simulink model "train_detection"  (R2024b)
settings: Solver=FixedStepAuto  StartTime=0.0  StopTime=simDuration  FixedStep=0.01  RelTol=1e-3
InitFcn:
  | breakp=[-1, -0.9, -0.8, -0.6, -0.4, -0.2, -0.1, 0, 0.1, 0.2, 0.4, 0.6, 0.8, 1];
  | 
  | splinenew =[-1, -0.92, -0.8, -0.50, -0.28, -0.12, -0.05, 0, 0.005, 0.01, 0.02, 0.025,0.03,0.035];
undefined symbols (not defined in the file or in its folder): Discrete, K, qbreak, Time
libraries: simulink x25, ctrlSharedLib x4, dspfdesign x2
(part 2 of 2)

== system train_detection/RIGHT_LEG/Pos and Vel normalized/Subsystem ==
  Angle : Inport
  Trigger : TriggerPort  VariantControl=Variant  PortDimensions=1
  Angle_min : Outport
  wires:
  Angle/1 -> Angle_min/1

== system train_detection/RIGHT_LEG/Pos and Vel normalized/Subsystem1 ==
  Velocity : Inport
  Trigger : TriggerPort  VariantControl=Variant  PortDimensions=1
  Vel_max : Outport
  wires:
  Velocity/1 -> Vel_max/1

== system train_detection/RIGHT_LEG/Pos and Vel normalized/Subsystem2 ==
  angle : Inport
  Trigger : TriggerPort  VariantControl=Variant  PortDimensions=1
  Angle_max : Outport
  wires:
  angle/1 -> Angle_max/1

== system train_detection/RIGHT_LEG/Pos and Vel normalized/Subsystem3 ==
  Velocity : Inport
  Trigger : TriggerPort  VariantControl=Variant  PortDimensions=1
  Vel_min : Outport
  wires:
  Velocity/1 -> Vel_min/1

== system train_detection/RIGHT_LEG/Pos and Vel normalized/Subsystem4 ==
  Clock : Inport
  angle : Inport  Port=2
  Trigger : TriggerPort  VariantControl=Variant  PortDimensions=1
  If : If  ShowElse=off
  If Action Subsystem : Subsystem  TreatAsAtomicUnit=on
  Angle_max : Outport
  wires:
  If/1 -> If Action Subsystem/Action
  angle/1 -> If Action Subsystem/2(angle), If/1
  If Action Subsystem/1(Angle_max) -> Angle_max/1  "angle_max"
  Clock/1 -> If Action Subsystem/1(Clock)  "clock"

== system train_detection/RIGHT_LEG/Pos and Vel normalized/Subsystem5 ==
  Angle : Inport
  Clock : Inport  Port=2
  Trigger : TriggerPort  VariantControl=Variant  PortDimensions=1
  If : If  IfExpression=u1 < 0  ShowElse=off
  If Action Subsystem : Subsystem  TreatAsAtomicUnit=on
  Angle_min : Outport
  wires:
  If/1 -> If Action Subsystem/Action
  Angle/1 -> If Action Subsystem/1(Angle), If/1
  If Action Subsystem/1(Angle_min) -> Angle_min/1  "angle_min"
  Clock/1 -> If Action Subsystem/2(Clock)  "clock"

== system train_detection/RIGHT_LEG/Pos and Vel normalized/Subsystem6 ==
  Velocity : Inport
  Clock : Inport  Port=2
  Trigger : TriggerPort  VariantControl=Variant  PortDimensions=1
  If : If  IfExpression=u1 < 0  ShowElse=off
  If Action Subsystem : Subsystem  TreatAsAtomicUnit=on
  Vel_min : Outport
  wires:
  If Action Subsystem/1(Vel_min) -> Vel_min/1  "vel_min"
  If/1 -> If Action Subsystem/Action
  Velocity/1 -> If Action Subsystem/1(Velocity), If/1
  Clock/1 -> If Action Subsystem/2(Clock)  "clock"

== system train_detection/RIGHT_LEG/Pos and Vel normalized/Subsystem7 ==
  Velocity : Inport
  Clock : Inport  Port=2
  Trigger : TriggerPort  VariantControl=Variant  PortDimensions=1
  If : If  ShowElse=off
  If Action Subsystem : Subsystem  TreatAsAtomicUnit=on
  Vel_max : Outport
  wires:
  If/1 -> If Action Subsystem/Action
  Velocity/1 -> If Action Subsystem/1(Velocity), If/1
  Clock/1 -> If Action Subsystem/2(Clock)  "clock"
  If Action Subsystem/1(Vel_max) -> Vel_max/1  "vel_max"

== system train_detection/RIGHT_LEG/Pos normalized/Subsystem ==
  Angle : Inport
  Clock : Inport  Port=2
  Trigger : TriggerPort  VariantControl=Variant  PortDimensions=1
  If : If  IfExpression=u1 < 0  ShowElse=off
  If Action Subsystem : Subsystem  TreatAsAtomicUnit=on
  Angle_min : Outport
  wires:
  If Action Subsystem/1(Angle_min) -> Angle_min/1  "angle_min"
  Clock/1 -> If Action Subsystem/2(Clock)  "clock"
  If/1 -> If Action Subsystem/Action
  Angle/1 -> If Action Subsystem/1(Angle), If/1

== system train_detection/RIGHT_LEG/Pos normalized/Subsystem2 ==
  Clock : Inport
  angle : Inport  Port=2
  Trigger : TriggerPort  VariantControl=Variant  PortDimensions=1
  If : If  ShowElse=off
  If Action Subsystem : Subsystem  TreatAsAtomicUnit=on
  Angle_out : Outport
  wires:
  If Action Subsystem/1(Angle_out) -> Angle_out/1  "angle_out"
  angle/1 -> If Action Subsystem/2(angle), If/1
  If/1 -> If Action Subsystem/Action
  Clock/1 -> If Action Subsystem/1(Clock)  "clock"

== system train_detection/RIGHT_LEG/Vel normalized/Subsystem1 ==
  Velocity : Inport
  Clock : Inport  Port=2
  Trigger : TriggerPort  VariantControl=Variant  PortDimensions=1
  If : If  ShowElse=off
  If Action Subsystem : Subsystem  TreatAsAtomicUnit=on
  Vel_max : Outport
  wires:
  If Action Subsystem/1(Vel_max) -> Vel_max/1  "vel_max"
  Velocity/1 -> If/1, If Action Subsystem/1(Velocity)
  If/1 -> If Action Subsystem/Action
  Clock/1 -> If Action Subsystem/2(Clock)  "clock"

== system train_detection/RIGHT_LEG/Vel normalized/Subsystem3 ==
  Velocity : Inport
  Clock : Inport  Port=2
  Trigger : TriggerPort  VariantControl=Variant  PortDimensions=1
  If : If  IfExpression=u1 < 0  ShowElse=off
  If Action Subsystem : Subsystem  TreatAsAtomicUnit=on
  Vel_min : Outport
  wires:
  If Action Subsystem/1(Vel_min) -> Vel_min/1  "vel_min"
  Clock/1 -> If Action Subsystem/2(Clock)  "clock"
  Velocity/1 -> If Action Subsystem/1(Velocity), If/1
  If/1 -> If Action Subsystem/Action

== system train_detection/RIGHT_LEG1/Pos and Vel normalized/Subsystem ==
  Angle : Inport
  Trigger : TriggerPort  VariantControl=Variant  PortDimensions=1
  Angle_min : Outport
  wires:
  Angle/1 -> Angle_min/1

== system train_detection/RIGHT_LEG1/Pos and Vel normalized/Subsystem1 ==
  Velocity : Inport
  Trigger : TriggerPort  VariantControl=Variant  PortDimensions=1
  Vel_max : Outport
  wires:
  Velocity/1 -> Vel_max/1

== system train_detection/RIGHT_LEG1/Pos and Vel normalized/Subsystem2 ==
  angle : Inport
  Trigger : TriggerPort  VariantControl=Variant  PortDimensions=1
  Angle_max : Outport
  wires:
  angle/1 -> Angle_max/1

== system train_detection/RIGHT_LEG1/Pos and Vel normalized/Subsystem3 ==
  Velocity : Inport
  Trigger : TriggerPort  VariantControl=Variant  PortDimensions=1
  Vel_min : Outport
  wires:
  Velocity/1 -> Vel_min/1

== system train_detection/RIGHT_LEG1/Pos and Vel normalized/Subsystem4 ==
  Clock : Inport
  angle : Inport  Port=2
  Trigger : TriggerPort  VariantControl=Variant  PortDimensions=1
  If : If  ShowElse=off
  If Action Subsystem : Subsystem  TreatAsAtomicUnit=on
  Angle_max : Outport
  wires:
  If/1 -> If Action Subsystem/Action
  angle/1 -> If Action Subsystem/2(angle), If/1
  If Action Subsystem/1(Angle_max) -> Angle_max/1  "angle_max"
  Clock/1 -> If Action Subsystem/1(Clock)  "clock"

== system train_detection/RIGHT_LEG1/Pos and Vel normalized/Subsystem5 ==
  Angle : Inport
  Clock : Inport  Port=2
  Trigger : TriggerPort  VariantControl=Variant  PortDimensions=1
  If : If  IfExpression=u1 < 0  ShowElse=off
  If Action Subsystem : Subsystem  TreatAsAtomicUnit=on
  Angle_min : Outport
  wires:
  If/1 -> If Action Subsystem/Action
  Angle/1 -> If Action Subsystem/1(Angle), If/1
  If Action Subsystem/1(Angle_min) -> Angle_min/1  "angle_min"
  Clock/1 -> If Action Subsystem/2(Clock)  "clock"

== system train_detection/RIGHT_LEG1/Pos and Vel normalized/Subsystem6 ==
  Velocity : Inport
  Clock : Inport  Port=2
  Trigger : TriggerPort  VariantControl=Variant  PortDimensions=1
  If : If  IfExpression=u1 < 0  ShowElse=off
  If Action Subsystem : Subsystem  TreatAsAtomicUnit=on
  Vel_min : Outport
  wires:
  If Action Subsystem/1(Vel_min) -> Vel_min/1  "vel_min"
  If/1 -> If Action Subsystem/Action
  Velocity/1 -> If Action Subsystem/1(Velocity), If/1
  Clock/1 -> If Action Subsystem/2(Clock)  "clock"

== system train_detection/RIGHT_LEG1/Pos and Vel normalized/Subsystem7 ==
  Velocity : Inport
  Clock : Inport  Port=2
  Trigger : TriggerPort  VariantControl=Variant  PortDimensions=1
  If : If  ShowElse=off
  If Action Subsystem : Subsystem  TreatAsAtomicUnit=on
  Vel_max : Outport
  wires:
  If/1 -> If Action Subsystem/Action
  Velocity/1 -> If Action Subsystem/1(Velocity), If/1
  Clock/1 -> If Action Subsystem/2(Clock)  "clock"
  If Action Subsystem/1(Vel_max) -> Vel_max/1  "vel_max"

== system train_detection/RIGHT_LEG1/Pos normalized/Subsystem ==
  Angle : Inport
  Clock : Inport  Port=2
  Trigger : TriggerPort  VariantControl=Variant  PortDimensions=1
  If : If  IfExpression=u1 < 0  ShowElse=off
  If Action Subsystem : Subsystem  TreatAsAtomicUnit=on
  Angle_min : Outport
  wires:
  If Action Subsystem/1(Angle_min) -> Angle_min/1  "angle_min"
  Clock/1 -> If Action Subsystem/2(Clock)  "clock"
  If/1 -> If Action Subsystem/Action
  Angle/1 -> If Action Subsystem/1(Angle), If/1

== system train_detection/RIGHT_LEG1/Pos normalized/Subsystem2 ==
  Clock : Inport
  angle : Inport  Port=2
  Trigger : TriggerPort  VariantControl=Variant  PortDimensions=1
  If : If  ShowElse=off
  If Action Subsystem : Subsystem  TreatAsAtomicUnit=on
  Angle_out : Outport
  wires:
  If Action Subsystem/1(Angle_out) -> Angle_out/1  "angle_out"
  angle/1 -> If Action Subsystem/2(angle), If/1
  If/1 -> If Action Subsystem/Action
  Clock/1 -> If Action Subsystem/1(Clock)  "clock"

== system train_detection/RIGHT_LEG1/Vel normalized/Subsystem1 ==
  Velocity : Inport
  Clock : Inport  Port=2
  Trigger : TriggerPort  VariantControl=Variant  PortDimensions=1
  If : If  ShowElse=off
  If Action Subsystem : Subsystem  TreatAsAtomicUnit=on
  Vel_max : Outport
  wires:
  If Action Subsystem/1(Vel_max) -> Vel_max/1  "vel_max"
  Velocity/1 -> If/1, If Action Subsystem/1(Velocity)
  If/1 -> If Action Subsystem/Action
  Clock/1 -> If Action Subsystem/2(Clock)  "clock"

== system train_detection/RIGHT_LEG1/Vel normalized/Subsystem3 ==
  Velocity : Inport
  Clock : Inport  Port=2
  Trigger : TriggerPort  VariantControl=Variant  PortDimensions=1
  If : If  IfExpression=u1 < 0  ShowElse=off
  If Action Subsystem : Subsystem  TreatAsAtomicUnit=on
  Vel_min : Outport
  wires:
  If Action Subsystem/1(Vel_min) -> Vel_min/1  "vel_min"
  Clock/1 -> If Action Subsystem/2(Clock)  "clock"
  Velocity/1 -> If Action Subsystem/1(Velocity), If/1
  If/1 -> If Action Subsystem/Action

== system train_detection/LEFT LEG/Pos and Vel normalized/Subsystem4/If Action Subsystem ==
  Clock : Inport
  angle : Inport  Port=2
  Action Port : ActionPort
  Compare To Constant1 : simulink/Logic and Bit Operations/Compare To Constant  relop=>=  const=0.3  OutDataTypeStr=boolean
  Enabled Subsystem : Subsystem  TreatAsAtomicUnit=on
  Memory : Memory  InheritSampleTime=on
  Subtract : Sum  Inputs=+-
  Zero-Order Hold : ZeroOrderHold  SampleTime=-1
  Angle_max : Outport
  wires:
  Subtract/1 -> Compare To Constant1/1  "diff"
  Compare To Constant1/1 -> Enabled Subsystem/Enable  "enable"
  Enabled Subsystem/1(angle_out) -> Angle_max/1  "angle_out"
  angle/1 -> Enabled Subsystem/1(angle_in)
  Clock/1 -> Zero-Order Hold/1  "clock"
  Zero-Order Hold/1 -> Subtract/1, Memory/1  "clock_ZOH"
  Memory/1 -> Subtract/2  "clock_memory"

== system train_detection/LEFT LEG/Pos and Vel normalized/Subsystem5/If Action Subsystem ==
  Angle : Inport
  Clock : Inport  Port=2
  Action Port : ActionPort
  Compare To Constant1 : simulink/Logic and Bit Operations/Compare To Constant  relop=>=  const=0.3  OutDataTypeStr=boolean
  Enabled Subsystem : Subsystem  TreatAsAtomicUnit=on
  Memory : Memory  InheritSampleTime=on
  Subtract : Sum  Inputs=+-
  Zero-Order Hold : ZeroOrderHold  SampleTime=-1
  Angle_min : Outport
  wires:
  Memory/1 -> Subtract/2  "clock_memory"
  Zero-Order Hold/1 -> Subtract/1, Memory/1  "clock_ZOH"
  Enabled Subsystem/1(angle_out) -> Angle_min/1  "angle_out"
  Compare To Constant1/1 -> Enabled Subsystem/Enable  "enable"
  Clock/1 -> Zero-Order Hold/1  "clock"
  Subtract/1 -> Compare To Constant1/1  "diff"
  Angle/1 -> Enabled Subsystem/1(angle_in)

== system train_detection/LEFT LEG/Pos and Vel normalized/Subsystem6/If Action Subsystem ==
  Velocity : Inport
  Clock : Inport  Port=2
  Action Port : ActionPort
  Compare To Constant1 : simulink/Logic and Bit Operations/Compare To Constant  relop=>=  const=0.3  OutDataTypeStr=boolean
  Enabled Subsystem : Subsystem  TreatAsAtomicUnit=on
  Memory : Memory  InheritSampleTime=on
  Subtract : Sum  Inputs=+-
  Zero-Order Hold : ZeroOrderHold  SampleTime=-1
  Vel_min : Outport
  wires:
  Enabled Subsystem/1(vel_out) -> Vel_min/1  "angle_out"
  Memory/1 -> Subtract/2  "clock_memory"
  Velocity/1 -> Enabled Subsystem/1(vel_in)
  Zero-Order Hold/1 -> Subtract/1, Memory/1  "clock_ZOH"
  Clock/1 -> Zero-Order Hold/1  "clock"
  Subtract/1 -> Compare To Constant1/1  "diff"
  Compare To Constant1/1 -> Enabled Subsystem/Enable  "enable"

== system train_detection/LEFT LEG/Pos and Vel normalized/Subsystem7/If Action Subsystem ==
  Velocity : Inport
  Clock : Inport  Port=2
  Action Port : ActionPort
  Compare To Constant1 : simulink/Logic and Bit Operations/Compare To Constant  relop=>=  const=0.3  OutDataTypeStr=boolean
  Enabled Subsystem : Subsystem  TreatAsAtomicUnit=on
  Memory : Memory  InheritSampleTime=on
  Subtract : Sum  Inputs=+-
  Zero-Order Hold : ZeroOrderHold  SampleTime=-1
  Vel_max : Outport
  wires:
  Memory/1 -> Subtract/2  "clock_memory"
  Compare To Constant1/1 -> Enabled Subsystem/Enable  "enable"
  Clock/1 -> Zero-Order Hold/1  "clock"
  Zero-Order Hold/1 -> Subtract/1, Memory/1  "clock_ZOH"
  Enabled Subsystem/1(vel_out) -> Vel_max/1  "angle_out"
  Subtract/1 -> Compare To Constant1/1  "diff"
  Velocity/1 -> Enabled Subsystem/1(vel_in)

== system train_detection/LEFT LEG1/Pos and Vel normalized/Subsystem4/If Action Subsystem ==
  Clock : Inport
  angle : Inport  Port=2
  Action Port : ActionPort
  Compare To Constant1 : simulink/Logic and Bit Operations/Compare To Constant  relop=>=  const=0.3  OutDataTypeStr=boolean
  Enabled Subsystem : Subsystem  TreatAsAtomicUnit=on
  Memory : Memory  InheritSampleTime=on
  Subtract : Sum  Inputs=+-
  Zero-Order Hold : ZeroOrderHold  SampleTime=-1
  Angle_max : Outport
  wires:
  Subtract/1 -> Compare To Constant1/1  "diff"
  Compare To Constant1/1 -> Enabled Subsystem/Enable  "enable"
  Enabled Subsystem/1(angle_out) -> Angle_max/1  "angle_out"
  angle/1 -> Enabled Subsystem/1(angle_in)
  Clock/1 -> Zero-Order Hold/1  "clock"
  Zero-Order Hold/1 -> Subtract/1, Memory/1  "clock_ZOH"
  Memory/1 -> Subtract/2  "clock_memory"

== system train_detection/LEFT LEG1/Pos and Vel normalized/Subsystem5/If Action Subsystem ==
  Angle : Inport
  Clock : Inport  Port=2
  Action Port : ActionPort
  Compare To Constant1 : simulink/Logic and Bit Operations/Compare To Constant  relop=>=  const=0.3  OutDataTypeStr=boolean
  Enabled Subsystem : Subsystem  TreatAsAtomicUnit=on
  Memory : Memory  InheritSampleTime=on
  Subtract : Sum  Inputs=+-
  Zero-Order Hold : ZeroOrderHold  SampleTime=-1
  Angle_min : Outport
  wires:
  Memory/1 -> Subtract/2  "clock_memory"
  Zero-Order Hold/1 -> Subtract/1, Memory/1  "clock_ZOH"
  Enabled Subsystem/1(angle_out) -> Angle_min/1  "angle_out"
  Compare To Constant1/1 -> Enabled Subsystem/Enable  "enable"
  Clock/1 -> Zero-Order Hold/1  "clock"
  Subtract/1 -> Compare To Constant1/1  "diff"
  Angle/1 -> Enabled Subsystem/1(angle_in)

== system train_detection/LEFT LEG1/Pos and Vel normalized/Subsystem6/If Action Subsystem ==
  Velocity : Inport
  Clock : Inport  Port=2
  Action Port : ActionPort
  Compare To Constant1 : simulink/Logic and Bit Operations/Compare To Constant  relop=>=  const=0.3  OutDataTypeStr=boolean
  Enabled Subsystem : Subsystem  TreatAsAtomicUnit=on
  Memory : Memory  InheritSampleTime=on
  Subtract : Sum  Inputs=+-
  Zero-Order Hold : ZeroOrderHold  SampleTime=-1
  Vel_min : Outport
  wires:
  Enabled Subsystem/1(vel_out) -> Vel_min/1  "angle_out"
  Memory/1 -> Subtract/2  "clock_memory"
  Velocity/1 -> Enabled Subsystem/1(vel_in)
  Zero-Order Hold/1 -> Subtract/1, Memory/1  "clock_ZOH"
  Clock/1 -> Zero-Order Hold/1  "clock"
  Subtract/1 -> Compare To Constant1/1  "diff"
  Compare To Constant1/1 -> Enabled Subsystem/Enable  "enable"

== system train_detection/LEFT LEG1/Pos and Vel normalized/Subsystem7/If Action Subsystem ==
  Velocity : Inport
  Clock : Inport  Port=2
  Action Port : ActionPort
  Compare To Constant1 : simulink/Logic and Bit Operations/Compare To Constant  relop=>=  const=0.3  OutDataTypeStr=boolean
  Enabled Subsystem : Subsystem  TreatAsAtomicUnit=on
  Memory : Memory  InheritSampleTime=on
  Subtract : Sum  Inputs=+-
  Zero-Order Hold : ZeroOrderHold  SampleTime=-1
  Vel_max : Outport
  wires:
  Memory/1 -> Subtract/2  "clock_memory"
  Compare To Constant1/1 -> Enabled Subsystem/Enable  "enable"
  Clock/1 -> Zero-Order Hold/1  "clock"
  Zero-Order Hold/1 -> Subtract/1, Memory/1  "clock_ZOH"
  Enabled Subsystem/1(vel_out) -> Vel_max/1  "angle_out"
  Subtract/1 -> Compare To Constant1/1  "diff"
  Velocity/1 -> Enabled Subsystem/1(vel_in)

== system train_detection/RIGHT_LEG/Pos and Vel normalized/Subsystem4/If Action Subsystem ==
  Clock : Inport
  angle : Inport  Port=2
  Action Port : ActionPort
  Compare To Constant1 : simulink/Logic and Bit Operations/Compare To Constant  relop=>=  const=0.3  OutDataTypeStr=boolean
  Enabled Subsystem : Subsystem  TreatAsAtomicUnit=on
  Memory : Memory  InheritSampleTime=on
  Subtract : Sum  Inputs=+-
  Zero-Order Hold : ZeroOrderHold  SampleTime=-1
  Angle_max : Outport
  wires:
  Subtract/1 -> Compare To Constant1/1  "diff"
  Compare To Constant1/1 -> Enabled Subsystem/Enable  "enable"
  Enabled Subsystem/1(angle_out) -> Angle_max/1  "angle_out"
  angle/1 -> Enabled Subsystem/1(angle_in)
  Clock/1 -> Zero-Order Hold/1  "clock"
  Zero-Order Hold/1 -> Subtract/1, Memory/1  "clock_ZOH"
  Memory/1 -> Subtract/2  "clock_memory"

== system train_detection/RIGHT_LEG/Pos and Vel normalized/Subsystem5/If Action Subsystem ==
  Angle : Inport
  Clock : Inport  Port=2
  Action Port : ActionPort
  Compare To Constant1 : simulink/Logic and Bit Operations/Compare To Constant  relop=>=  const=0.3  OutDataTypeStr=boolean
  Enabled Subsystem : Subsystem  TreatAsAtomicUnit=on
  Memory : Memory  InheritSampleTime=on
  Subtract : Sum  Inputs=+-
  Zero-Order Hold : ZeroOrderHold  SampleTime=-1
  Angle_min : Outport
  wires:
  Memory/1 -> Subtract/2  "clock_memory"
  Zero-Order Hold/1 -> Subtract/1, Memory/1  "clock_ZOH"
  Enabled Subsystem/1(angle_out) -> Angle_min/1  "angle_out"
  Compare To Constant1/1 -> Enabled Subsystem/Enable  "enable"
  Clock/1 -> Zero-Order Hold/1  "clock"
  Subtract/1 -> Compare To Constant1/1  "diff"
  Angle/1 -> Enabled Subsystem/1(angle_in)

== system train_detection/RIGHT_LEG/Pos and Vel normalized/Subsystem6/If Action Subsystem ==
  Velocity : Inport
  Clock : Inport  Port=2
  Action Port : ActionPort
  Compare To Constant1 : simulink/Logic and Bit Operations/Compare To Constant  relop=>=  const=0.3  OutDataTypeStr=boolean
  Enabled Subsystem : Subsystem  TreatAsAtomicUnit=on
  Memory : Memory  InheritSampleTime=on
  Subtract : Sum  Inputs=+-
  Zero-Order Hold : ZeroOrderHold  SampleTime=-1
  Vel_min : Outport
  wires:
  Enabled Subsystem/1(vel_out) -> Vel_min/1  "angle_out"
  Memory/1 -> Subtract/2  "clock_memory"
  Velocity/1 -> Enabled Subsystem/1(vel_in)
  Zero-Order Hold/1 -> Subtract/1, Memory/1  "clock_ZOH"
  Clock/1 -> Zero-Order Hold/1  "clock"
  Subtract/1 -> Compare To Constant1/1  "diff"
  Compare To Constant1/1 -> Enabled Subsystem/Enable  "enable"

== system train_detection/RIGHT_LEG/Pos and Vel normalized/Subsystem7/If Action Subsystem ==
  Velocity : Inport
  Clock : Inport  Port=2
  Action Port : ActionPort
  Compare To Constant1 : simulink/Logic and Bit Operations/Compare To Constant  relop=>=  const=0.3  OutDataTypeStr=boolean
  Enabled Subsystem : Subsystem  TreatAsAtomicUnit=on
  Memory : Memory  InheritSampleTime=on
  Subtract : Sum  Inputs=+-
  Zero-Order Hold : ZeroOrderHold  SampleTime=-1
  Vel_max : Outport
  wires:
  Memory/1 -> Subtract/2  "clock_memory"
  Compare To Constant1/1 -> Enabled Subsystem/Enable  "enable"
  Clock/1 -> Zero-Order Hold/1  "clock"
  Zero-Order Hold/1 -> Subtract/1, Memory/1  "clock_ZOH"
  Enabled Subsystem/1(vel_out) -> Vel_max/1  "angle_out"
  Subtract/1 -> Compare To Constant1/1  "diff"
  Velocity/1 -> Enabled Subsystem/1(vel_in)

== system train_detection/RIGHT_LEG/Pos normalized/Subsystem/If Action Subsystem ==
  Angle : Inport
  Clock : Inport  Port=2
  Action Port : ActionPort  ActionPortLabel=if(u1 < 0)
  Compare To Constant1 : simulink/Logic and Bit Operations/Compare To Constant  relop=>=  const=0.3  OutDataTypeStr=boolean
  Enabled Subsystem : Subsystem  TreatAsAtomicUnit=on
  Memory : Memory  InheritSampleTime=on
  Subtract : Sum  Inputs=+-
  Zero-Order Hold : ZeroOrderHold  SampleTime=-1
  Angle_min : Outport
  wires:
  Enabled Subsystem/1(angle_out) -> Angle_min/1  "angle_out"
  Clock/1 -> Zero-Order Hold/1  "clock"
  Subtract/1 -> Compare To Constant1/1  "diff"
  Angle/1 -> Enabled Subsystem/1(angle_in)
  Compare To Constant1/1 -> Enabled Subsystem/Enable  "enable"
  Zero-Order Hold/1 -> Subtract/1, Memory/1  "clock_ZOH"
  Memory/1 -> Subtract/2  "clock_memory"

== system train_detection/RIGHT_LEG/Pos normalized/Subsystem2/If Action Subsystem ==
  Clock : Inport
  angle : Inport  Port=2
  Action Port : ActionPort  ActionPortLabel=if(u1 > 0)
  Compare To Constant1 : simulink/Logic and Bit Operations/Compare To Constant  relop=>=  const=0.3  OutDataTypeStr=boolean
  Enabled Subsystem : Subsystem  TreatAsAtomicUnit=on
  Memory : Memory  InheritSampleTime=on
  Subtract : Sum  Inputs=+-
  Zero-Order Hold : ZeroOrderHold  SampleTime=-1
  Angle_out : Outport
  wires:
  Zero-Order Hold/1 -> Memory/1, Subtract/1  "clock_ZOH"
  Memory/1 -> Subtract/2  "clock_memory"
  Subtract/1 -> Compare To Constant1/1  "diff"
  Enabled Subsystem/1(angle_out) -> Angle_out/1  "angle_out"
  Clock/1 -> Zero-Order Hold/1  "clock"
  angle/1 -> Enabled Subsystem/1(angle_in)
  Compare To Constant1/1 -> Enabled Subsystem/Enable  "enable"

== system train_detection/RIGHT_LEG/Vel normalized/Subsystem1/If Action Subsystem ==
  Velocity : Inport
  Clock : Inport  Port=2
  Action Port : ActionPort  ActionPortLabel=if(u1 > 0)
  Compare To Constant1 : simulink/Logic and Bit Operations/Compare To Constant  relop=>=  const=0.3  OutDataTypeStr=boolean
  Enabled Subsystem : Subsystem  TreatAsAtomicUnit=on
  Memory : Memory  InheritSampleTime=on
  Subtract : Sum  Inputs=+-
  Zero-Order Hold : ZeroOrderHold  SampleTime=-1
  Vel_max : Outport
  wires:
  Clock/1 -> Zero-Order Hold/1  "clock"
  Memory/1 -> Subtract/2  "clock_memory"
  Enabled Subsystem/1(vel_out) -> Vel_max/1  "angle_out"
  Zero-Order Hold/1 -> Subtract/1, Memory/1  "clock_ZOH"
  Compare To Constant1/1 -> Enabled Subsystem/Enable  "enable"
  Subtract/1 -> Compare To Constant1/1  "diff"
  Velocity/1 -> Enabled Subsystem/1(vel_in)

== system train_detection/RIGHT_LEG/Vel normalized/Subsystem3/If Action Subsystem ==
  Velocity : Inport
  Clock : Inport  Port=2
  Action Port : ActionPort  ActionPortLabel=if(u1 < 0)
  Compare To Constant1 : simulink/Logic and Bit Operations/Compare To Constant  relop=>=  const=0.3  OutDataTypeStr=boolean
  Enabled Subsystem : Subsystem  TreatAsAtomicUnit=on
  Memory : Memory  InheritSampleTime=on
  Subtract : Sum  Inputs=+-
  Zero-Order Hold : ZeroOrderHold  SampleTime=-1
  Vel_min : Outport
  wires:
  Velocity/1 -> Enabled Subsystem/1(vel_in)
  Compare To Constant1/1 -> Enabled Subsystem/Enable  "enable"
  Clock/1 -> Zero-Order Hold/1  "clock"
  Subtract/1 -> Compare To Constant1/1  "diff"
  Zero-Order Hold/1 -> Subtract/1, Memory/1  "clock_ZOH"
  Memory/1 -> Subtract/2  "clock_memory"
  Enabled Subsystem/1(vel_out) -> Vel_min/1  "angle_out"

== system train_detection/RIGHT_LEG1/Pos and Vel normalized/Subsystem4/If Action Subsystem ==
  Clock : Inport
  angle : Inport  Port=2
  Action Port : ActionPort
  Compare To Constant1 : simulink/Logic and Bit Operations/Compare To Constant  relop=>=  const=0.3  OutDataTypeStr=boolean
  Enabled Subsystem : Subsystem  TreatAsAtomicUnit=on
  Memory : Memory  InheritSampleTime=on
  Subtract : Sum  Inputs=+-
  Zero-Order Hold : ZeroOrderHold  SampleTime=-1
  Angle_max : Outport
  wires:
  Subtract/1 -> Compare To Constant1/1  "diff"
  Compare To Constant1/1 -> Enabled Subsystem/Enable  "enable"
  Enabled Subsystem/1(angle_out) -> Angle_max/1  "angle_out"
  angle/1 -> Enabled Subsystem/1(angle_in)
  Clock/1 -> Zero-Order Hold/1  "clock"
  Zero-Order Hold/1 -> Subtract/1, Memory/1  "clock_ZOH"
  Memory/1 -> Subtract/2  "clock_memory"

== system train_detection/RIGHT_LEG1/Pos and Vel normalized/Subsystem5/If Action Subsystem ==
  Angle : Inport
  Clock : Inport  Port=2
  Action Port : ActionPort
  Compare To Constant1 : simulink/Logic and Bit Operations/Compare To Constant  relop=>=  const=0.3  OutDataTypeStr=boolean
  Enabled Subsystem : Subsystem  TreatAsAtomicUnit=on
  Memory : Memory  InheritSampleTime=on
  Subtract : Sum  Inputs=+-
  Zero-Order Hold : ZeroOrderHold  SampleTime=-1
  Angle_min : Outport
  wires:
  Memory/1 -> Subtract/2  "clock_memory"
  Zero-Order Hold/1 -> Subtract/1, Memory/1  "clock_ZOH"
  Enabled Subsystem/1(angle_out) -> Angle_min/1  "angle_out"
  Compare To Constant1/1 -> Enabled Subsystem/Enable  "enable"
  Clock/1 -> Zero-Order Hold/1  "clock"
  Subtract/1 -> Compare To Constant1/1  "diff"
  Angle/1 -> Enabled Subsystem/1(angle_in)

== system train_detection/RIGHT_LEG1/Pos and Vel normalized/Subsystem6/If Action Subsystem ==
  Velocity : Inport
  Clock : Inport  Port=2
  Action Port : ActionPort
  Compare To Constant1 : simulink/Logic and Bit Operations/Compare To Constant  relop=>=  const=0.3  OutDataTypeStr=boolean
  Enabled Subsystem : Subsystem  TreatAsAtomicUnit=on
  Memory : Memory  InheritSampleTime=on
  Subtract : Sum  Inputs=+-
  Zero-Order Hold : ZeroOrderHold  SampleTime=-1
  Vel_min : Outport
  wires:
  Enabled Subsystem/1(vel_out) -> Vel_min/1  "angle_out"
  Memory/1 -> Subtract/2  "clock_memory"
  Velocity/1 -> Enabled Subsystem/1(vel_in)
  Zero-Order Hold/1 -> Subtract/1, Memory/1  "clock_ZOH"
  Clock/1 -> Zero-Order Hold/1  "clock"
  Subtract/1 -> Compare To Constant1/1  "diff"
  Compare To Constant1/1 -> Enabled Subsystem/Enable  "enable"

== system train_detection/RIGHT_LEG1/Pos and Vel normalized/Subsystem7/If Action Subsystem ==
  Velocity : Inport
  Clock : Inport  Port=2
  Action Port : ActionPort
  Compare To Constant1 : simulink/Logic and Bit Operations/Compare To Constant  relop=>=  const=0.3  OutDataTypeStr=boolean
  Enabled Subsystem : Subsystem  TreatAsAtomicUnit=on
  Memory : Memory  InheritSampleTime=on
  Subtract : Sum  Inputs=+-
  Zero-Order Hold : ZeroOrderHold  SampleTime=-1
  Vel_max : Outport
  wires:
  Memory/1 -> Subtract/2  "clock_memory"
  Compare To Constant1/1 -> Enabled Subsystem/Enable  "enable"
  Clock/1 -> Zero-Order Hold/1  "clock"
  Zero-Order Hold/1 -> Subtract/1, Memory/1  "clock_ZOH"
  Enabled Subsystem/1(vel_out) -> Vel_max/1  "angle_out"
  Subtract/1 -> Compare To Constant1/1  "diff"
  Velocity/1 -> Enabled Subsystem/1(vel_in)

== system train_detection/RIGHT_LEG1/Pos normalized/Subsystem/If Action Subsystem ==
  Angle : Inport
  Clock : Inport  Port=2
  Action Port : ActionPort
  Compare To Constant1 : simulink/Logic and Bit Operations/Compare To Constant  relop=>=  const=0.3  OutDataTypeStr=boolean
  Enabled Subsystem : Subsystem  TreatAsAtomicUnit=on
  Memory : Memory  InheritSampleTime=on
  Subtract : Sum  Inputs=+-
  Zero-Order Hold : ZeroOrderHold  SampleTime=-1
  Angle_min : Outport
  wires:
  Enabled Subsystem/1(angle_out) -> Angle_min/1  "angle_out"
  Clock/1 -> Zero-Order Hold/1  "clock"
  Subtract/1 -> Compare To Constant1/1  "diff"
  Angle/1 -> Enabled Subsystem/1(angle_in)
  Compare To Constant1/1 -> Enabled Subsystem/Enable  "enable"
  Zero-Order Hold/1 -> Subtract/1, Memory/1  "clock_ZOH"
  Memory/1 -> Subtract/2  "clock_memory"

== system train_detection/RIGHT_LEG1/Pos normalized/Subsystem2/If Action Subsystem ==
  Clock : Inport
  angle : Inport  Port=2
  Action Port : ActionPort
  Compare To Constant1 : simulink/Logic and Bit Operations/Compare To Constant  relop=>=  const=0.3  OutDataTypeStr=boolean
  Enabled Subsystem : Subsystem  TreatAsAtomicUnit=on
  Memory : Memory  InheritSampleTime=on
  Subtract : Sum  Inputs=+-
  Zero-Order Hold : ZeroOrderHold  SampleTime=-1
  Angle_out : Outport
  wires:
  Zero-Order Hold/1 -> Memory/1, Subtract/1  "clock_ZOH"
  Memory/1 -> Subtract/2  "clock_memory"
  Subtract/1 -> Compare To Constant1/1  "diff"
  Enabled Subsystem/1(angle_out) -> Angle_out/1  "angle_out"
  Clock/1 -> Zero-Order Hold/1  "clock"
  angle/1 -> Enabled Subsystem/1(angle_in)
  Compare To Constant1/1 -> Enabled Subsystem/Enable  "enable"

== system train_detection/RIGHT_LEG1/Vel normalized/Subsystem1/If Action Subsystem ==
  Velocity : Inport
  Clock : Inport  Port=2
  Action Port : ActionPort
  Compare To Constant1 : simulink/Logic and Bit Operations/Compare To Constant  relop=>=  const=0.3  OutDataTypeStr=boolean
  Enabled Subsystem : Subsystem  TreatAsAtomicUnit=on
  Memory : Memory  InheritSampleTime=on
  Subtract : Sum  Inputs=+-
  Zero-Order Hold : ZeroOrderHold  SampleTime=-1
  Vel_max : Outport
  wires:
  Clock/1 -> Zero-Order Hold/1  "clock"
  Memory/1 -> Subtract/2  "clock_memory"
  Enabled Subsystem/1(vel_out) -> Vel_max/1  "angle_out"
  Zero-Order Hold/1 -> Subtract/1, Memory/1  "clock_ZOH"
  Compare To Constant1/1 -> Enabled Subsystem/Enable  "enable"
  Subtract/1 -> Compare To Constant1/1  "diff"
  Velocity/1 -> Enabled Subsystem/1(vel_in)

== system train_detection/RIGHT_LEG1/Vel normalized/Subsystem3/If Action Subsystem ==
  Velocity : Inport
  Clock : Inport  Port=2
  Action Port : ActionPort
  Compare To Constant1 : simulink/Logic and Bit Operations/Compare To Constant  relop=>=  const=0.3  OutDataTypeStr=boolean
  Enabled Subsystem : Subsystem  TreatAsAtomicUnit=on
  Memory : Memory  InheritSampleTime=on
  Subtract : Sum  Inputs=+-
  Zero-Order Hold : ZeroOrderHold  SampleTime=-1
  Vel_min : Outport
  wires:
  Velocity/1 -> Enabled Subsystem/1(vel_in)
  Compare To Constant1/1 -> Enabled Subsystem/Enable  "enable"
  Clock/1 -> Zero-Order Hold/1  "clock"
  Subtract/1 -> Compare To Constant1/1  "diff"
  Zero-Order Hold/1 -> Subtract/1, Memory/1  "clock_ZOH"
  Memory/1 -> Subtract/2  "clock_memory"
  Enabled Subsystem/1(vel_out) -> Vel_min/1  "angle_out"

== system train_detection/LEFT LEG/Pos and Vel normalized/Subsystem4/If Action Subsystem/Enabled Subsystem ==
  angle_in : Inport
  Enable : EnablePort
  angle_out : Outport
  wires:
  angle_in/1 -> angle_out/1

== system train_detection/LEFT LEG/Pos and Vel normalized/Subsystem5/If Action Subsystem/Enabled Subsystem ==
  angle_in : Inport
  Enable : EnablePort
  angle_out : Outport
  wires:
  angle_in/1 -> angle_out/1

== system train_detection/LEFT LEG/Pos and Vel normalized/Subsystem6/If Action Subsystem/Enabled Subsystem ==
  vel_in : Inport
  Enable : EnablePort
  vel_out : Outport
  wires:
  vel_in/1 -> vel_out/1

== system train_detection/LEFT LEG/Pos and Vel normalized/Subsystem7/If Action Subsystem/Enabled Subsystem ==
  vel_in : Inport
  Enable : EnablePort
  vel_out : Outport
  wires:
  vel_in/1 -> vel_out/1

== system train_detection/LEFT LEG1/Pos and Vel normalized/Subsystem4/If Action Subsystem/Enabled Subsystem ==
  angle_in : Inport
  Enable : EnablePort
  angle_out : Outport
  wires:
  angle_in/1 -> angle_out/1

== system train_detection/LEFT LEG1/Pos and Vel normalized/Subsystem5/If Action Subsystem/Enabled Subsystem ==
  angle_in : Inport
  Enable : EnablePort
  angle_out : Outport
  wires:
  angle_in/1 -> angle_out/1

== system train_detection/LEFT LEG1/Pos and Vel normalized/Subsystem6/If Action Subsystem/Enabled Subsystem ==
  vel_in : Inport
  Enable : EnablePort
  vel_out : Outport
  wires:
  vel_in/1 -> vel_out/1

== system train_detection/LEFT LEG1/Pos and Vel normalized/Subsystem7/If Action Subsystem/Enabled Subsystem ==
  vel_in : Inport
  Enable : EnablePort
  vel_out : Outport
  wires:
  vel_in/1 -> vel_out/1

== system train_detection/RIGHT_LEG/Pos and Vel normalized/Subsystem4/If Action Subsystem/Enabled Subsystem ==
  angle_in : Inport
  Enable : EnablePort
  angle_out : Outport
  wires:
  angle_in/1 -> angle_out/1

== system train_detection/RIGHT_LEG/Pos and Vel normalized/Subsystem5/If Action Subsystem/Enabled Subsystem ==
  angle_in : Inport
  Enable : EnablePort
  angle_out : Outport
  wires:
  angle_in/1 -> angle_out/1

== system train_detection/RIGHT_LEG/Pos and Vel normalized/Subsystem6/If Action Subsystem/Enabled Subsystem ==
  vel_in : Inport
  Enable : EnablePort
  vel_out : Outport
  wires:
  vel_in/1 -> vel_out/1

== system train_detection/RIGHT_LEG/Pos and Vel normalized/Subsystem7/If Action Subsystem/Enabled Subsystem ==
  vel_in : Inport
  Enable : EnablePort
  vel_out : Outport
  wires:
  vel_in/1 -> vel_out/1

== system train_detection/RIGHT_LEG/Pos normalized/Subsystem/If Action Subsystem/Enabled Subsystem ==
  angle_in : Inport
  Enable : EnablePort
  angle_out : Outport
  wires:
  angle_in/1 -> angle_out/1

== system train_detection/RIGHT_LEG/Pos normalized/Subsystem2/If Action Subsystem/Enabled Subsystem ==
  angle_in : Inport
  Enable : EnablePort
  angle_out : Outport
  wires:
  angle_in/1 -> angle_out/1

== system train_detection/RIGHT_LEG/Vel normalized/Subsystem1/If Action Subsystem/Enabled Subsystem ==
  vel_in : Inport
  Enable : EnablePort
  vel_out : Outport
  wires:
  vel_in/1 -> vel_out/1

== system train_detection/RIGHT_LEG/Vel normalized/Subsystem3/If Action Subsystem/Enabled Subsystem ==
  vel_in : Inport
  Enable : EnablePort
  vel_out : Outport
  wires:
  vel_in/1 -> vel_out/1

== system train_detection/RIGHT_LEG1/Pos and Vel normalized/Subsystem4/If Action Subsystem/Enabled Subsystem ==
  angle_in : Inport
  Enable : EnablePort
  angle_out : Outport
  wires:
  angle_in/1 -> angle_out/1

== system train_detection/RIGHT_LEG1/Pos and Vel normalized/Subsystem5/If Action Subsystem/Enabled Subsystem ==
  angle_in : Inport
  Enable : EnablePort
  angle_out : Outport
  wires:
  angle_in/1 -> angle_out/1

== system train_detection/RIGHT_LEG1/Pos and Vel normalized/Subsystem6/If Action Subsystem/Enabled Subsystem ==
  vel_in : Inport
  Enable : EnablePort
  vel_out : Outport
  wires:
  vel_in/1 -> vel_out/1

== system train_detection/RIGHT_LEG1/Pos and Vel normalized/Subsystem7/If Action Subsystem/Enabled Subsystem ==
  vel_in : Inport
  Enable : EnablePort
  vel_out : Outport
  wires:
  vel_in/1 -> vel_out/1

== system train_detection/RIGHT_LEG1/Pos normalized/Subsystem/If Action Subsystem/Enabled Subsystem ==
  angle_in : Inport
  Enable : EnablePort
  angle_out : Outport
  wires:
  angle_in/1 -> angle_out/1

== system train_detection/RIGHT_LEG1/Pos normalized/Subsystem2/If Action Subsystem/Enabled Subsystem ==
  angle_in : Inport
  Enable : EnablePort
  angle_out : Outport
  wires:
  angle_in/1 -> angle_out/1

== system train_detection/RIGHT_LEG1/Vel normalized/Subsystem1/If Action Subsystem/Enabled Subsystem ==
  vel_in : Inport
  Enable : EnablePort
  vel_out : Outport
  wires:
  vel_in/1 -> vel_out/1

== system train_detection/RIGHT_LEG1/Vel normalized/Subsystem3/If Action Subsystem/Enabled Subsystem ==
  vel_in : Inport
  Enable : EnablePort
  vel_out : Outport
  wires:
  vel_in/1 -> vel_out/1

== matlab function train_detection/IMUs/KF_L ==
  data: angle_meas input; angle_filt output; gyro_meas input; dt input; omega_filt output; bias_filt output; Qangle input; Qvel input; Qbias input; Rangle input; Rvel input
function [angle_filt, omega_filt, bias_filt] = KF_IMU(angle_meas, gyro_meas, dt, Qangle, Qvel, Qbias, Rangle, Rvel)
% Kalman Filter for [angle, omega, bias]

persistent x P F H Q R
if isempty(x)
    % initial state
    x = [angle_meas; gyro_meas; 0];
    
    % initial covariance
    P = diag([1e-2 1e-2 1e-3]);

    % system matrix
    F = [1 dt 0;
         0 1  0;
         0 0  1];

    % measurement matrix
    H = [1 0 0;
         0 1 1];

    % process noise
    %Q = diag([1e-5 1e-4 1e-7]);%[1e-5 1e-3 1e-7];
    Q = diag([Qangle Qvel Qbias]);

    % measurement noise
    %R = diag([8e-3 5e-1]);%[1e-2 1e-4];
    R = diag([Rangle Rvel]);

    %Q1(Q_θθ):	Angle process noise	(small: keeps angle smooth)
    %Q2(Q_ωω):	Velocity process noise	(small: slower velocity changes to suppress spikes)
    %Q3(Q_bb):	Gyro bias process noise (small: keeps bias stable (velocity smoother but bias offset for drift less responsive))
    %R1(R_θ):	Angle measurement noise	(small: trusts angle strongly, helps smooth velocity)
    %R2(R_ω):	Gyro measurement noise	(higher: ignores small/high spikes from gyro)
end

%% PREDICT
x = F * x;
P = F * P * F.' + Q;

%% UPDATE
z = [angle_meas; gyro_meas];
S = H * P * H.' + R;
K = P * H.' / S;

y = z - H*x;      % residual
x = x + K * y;
P = (eye(3) - K*H) * P;

angle_filt = x(1);
omega_filt = x(2);
bias_filt  = x(3);

== matlab function train_detection/IMUs/Kalman_Filter ==
  data: y input; x_hat output
function x_hat = kalman_hip(y)
% y: measured angle (scalar)
% x_hat: [theta_hat; theta_dot_hat]

persistent A C Q R P x
persistent initialized

Ts = 0.01; % sample time

if isempty(initialized)
    A = [1 Ts; 0 1];
    C = [1 0];

    % Tune these:
    Q = [1e-6      0;
        0      5e-3];   % more process noise on velocity state
    R = 9e-4;            % measurement noise variance (rad^2)

    P = eye(2);        % initial covariance
    x = [0; 0];        % initial state estimate
    initialized = true;
end

% Prediction
x_pred = A * x;
P_pred = A * P * A' + Q;

% Innovation
y_pred = C * x_pred;
e = y - y_pred;  % innovation

S = C * P_pred * C' + R;
K = P_pred * C' / S;  % Kalman gain (2x1)

% Update
x = x_pred + K * e;
P = (eye(2) - K * C) * P_pred;

x_hat = x;

== matlab function train_detection/IMUs/KF_R ==
  data: angle_meas input; angle_filt output; gyro_meas input; dt input; omega_filt output; bias_filt output; Qangle input; Qvel input; Qbias input; Rangle input; Rvel input
function [angle_filt, omega_filt, bias_filt] = KF_IMU(angle_meas, gyro_meas, dt, Qangle, Qvel, Qbias, Rangle, Rvel)
% Kalman Filter for [angle, omega, bias]

persistent x P F H Q R
if isempty(x)
    % initial state
    x = [angle_meas; gyro_meas; 0];
    
    % initial covariance
    P = diag([1e-2 1e-2 1e-3]);

    % system matrix
    F = [1 dt 0;
         0 1  0;
         0 0  1];

    % measurement matrix
    H = [1 0 0;
         0 1 1];

    % process noise
    %Q = diag([1e-5 1e-4 1e-7]);%[1e-5 1e-3 1e-7];
    Q = diag([Qangle Qvel Qbias]);

    % measurement noise
    %R = diag([8e-3 5e-1]);%[1e-2 1e-4];
    R = diag([Rangle Rvel]);

    %Q1(Q_θθ):	Angle process noise	(small: keeps angle smooth)
    %Q2(Q_ωω):	Velocity process noise	(small: slower velocity changes to suppress spikes)
    %Q3(Q_bb):	Gyro bias process noise (small: keeps bias stable (velocity smoother but bias offset for drift less responsive))
    %R1(R_θ):	Angle measurement noise	(small: trusts angle strongly, helps smooth velocity)
    %R2(R_ω):	Gyro measurement noise	(higher: ignores small/high spikes from gyro)
end

%% PREDICT
x = F * x;
P = F * P * F.' + Q;

%% UPDATE
z = [angle_meas; gyro_meas];
S = H * P * H.' + R;
K = P * H.' / S;

y = z - H*x;      % residual
x = x + K * y;
P = (eye(3) - K*H) * P;

angle_filt = x(1);
omega_filt = x(2);
bias_filt  = x(3);

== stateflow chart train_detection/RIGHT_LEG/Pos and Vel normalized/Chart ==
  settings: updateMethod=DISCRETE  sampleTime=0.01
  state Expect_Vel_Max
    entry: valid_ang_min = 1;
    during:
    valid_vel_max = 0;
    valid_vel_min = 0;
    valid_ang_max = 0;
    valid_ang_min = 0;
  state Expect_Ang_Max
    entry: valid_vel_max = 1;
    during:
    valid_vel_max = 0;
    valid_vel_min = 0;
    valid_ang_max = 0;
    valid_ang_min = 0;
  state Resync
    valid_vel_max = 0;
    valid_vel_min = 0;
    valid_ang_max = 0;
    valid_ang_min = 0;
  state Expect_Vel_Min
    entry: valid_ang_max = 1;
    during:
    valid_vel_max = 0;
    valid_vel_min = 0;
    valid_ang_max = 0;
    valid_ang_min = 0;
  state Expect_Ang_Min
    entry: valid_vel_min = 1;
    during:
    valid_vel_max = 0;
    valid_vel_min = 0;
    valid_ang_max = 0;
    valid_ang_min = 0;
  Expect_Vel_Max -> Expect_Ang_Max [order 1] : [vel_max && after(Tmin, tick) && before(Tmax, tick) && vel > 0]
  Resync -> Expect_Ang_Max [order 1] : [vel_max && vel > 0]
  Expect_Vel_Max -> Resync [order 2] : [after(Tmax, tick)]
  Expect_Ang_Max -> Resync [order 2] : [after(Tmax, tick)]
  Expect_Ang_Max -> Expect_Vel_Min [order 1] : [ang_max && after(Tmin, tick) && before(Tmax, tick) && angle > 0]
  Expect_Ang_Min -> Expect_Vel_Max [order 2] : [ang_min && after(Tmin, tick) && before(Tmax, tick) && angle < 0]
  Resync -> Expect_Vel_Max [order 3] : [ang_min && angle < 0]
  Expect_Vel_Min -> Resync [order 1] : [after(Tmax, tick)]
  (default) -> Resync : {valid_vel_max = 0;
      | valid_vel_min = 0;
      | valid_ang_max = 0;
      | valid_ang_min = 0;}
  Resync -> Expect_Vel_Min [order 4] : [ang_max && angle > 0]
  Expect_Ang_Min -> Resync [order 1] : [after(Tmax, tick)]
  Resync -> Expect_Ang_Min [order 2] : [vel_min && vel < 0]
  Expect_Vel_Min -> Expect_Ang_Min [order 2] : [vel_min && after(Tmin, tick) && before(Tmax, tick) && vel < 0]
  data: ang_max input; vel_min input; vel_max input; ang_min input; valid_vel_max output; valid_vel_min output; valid_ang_max output; valid_ang_min output; Tmin local double =0; Tmax local double =60; vel input; angle input

== stateflow chart train_detection/LEFT LEG1/Pos and Vel normalized/Chart ==
  settings: updateMethod=DISCRETE  sampleTime=0.01
  state Expect_Vel_Max
    entry: valid_ang_min = 1;
    during:
    valid_vel_max = 0;
    valid_vel_min = 0;
    valid_ang_max = 0;
    valid_ang_min = 0;
  state Expect_Ang_Max
    entry: valid_vel_max = 1;
    during:
    valid_vel_max = 0;
    valid_vel_min = 0;
    valid_ang_max = 0;
    valid_ang_min = 0;
  state Resync
    valid_vel_max = 0;
    valid_vel_min = 0;
    valid_ang_max = 0;
    valid_ang_min = 0;
  state Expect_Vel_Min
    entry: valid_ang_max = 1;
    during:
    valid_vel_max = 0;
    valid_vel_min = 0;
    valid_ang_max = 0;
    valid_ang_min = 0;
  state Expect_Ang_Min
    entry: valid_vel_min = 1;
    during:
    valid_vel_max = 0;
    valid_vel_min = 0;
    valid_ang_max = 0;
    valid_ang_min = 0;
  Expect_Vel_Max -> Expect_Ang_Max [order 1] : [vel_max && after(Tmin, tick) && before(Tmax, tick) && vel > 0]
  Resync -> Expect_Ang_Max [order 1] : [vel_max && vel > 0]
  Expect_Vel_Max -> Resync [order 2] : [after(Tmax, tick)]
  Expect_Ang_Max -> Resync [order 2] : [after(Tmax, tick)]
  Expect_Ang_Max -> Expect_Vel_Min [order 1] : [ang_max && after(Tmin, tick) && before(Tmax, tick) && angle > 0]
  Expect_Ang_Min -> Expect_Vel_Max [order 2] : [ang_min && after(Tmin, tick) && before(Tmax, tick) && angle < 0]
  Resync -> Expect_Vel_Max [order 3] : [ang_min && angle < 0]
  Expect_Vel_Min -> Resync [order 1] : [after(Tmax, tick)]
  (default) -> Resync : {valid_vel_max = 0;
      | valid_vel_min = 0;
      | valid_ang_max = 0;
      | valid_ang_min = 0;}
  Resync -> Expect_Vel_Min [order 4] : [ang_max && angle > 0]
  Expect_Ang_Min -> Resync [order 1] : [after(Tmax, tick)]
  Resync -> Expect_Ang_Min [order 2] : [vel_min && vel < 0]
  Expect_Vel_Min -> Expect_Ang_Min [order 2] : [vel_min && after(Tmin, tick) && before(Tmax, tick) && vel < 0]
  data: ang_max input; vel_min input; vel_max input; ang_min input; valid_vel_max output; valid_vel_min output; valid_ang_max output; valid_ang_min output; Tmin local double =0; Tmax local double =60; vel input; angle input

== matlab function train_detection/MATLAB Function ==
  data: Gait_phaseR input; Gait_phaseL input; STOPR input; STOPL input; output output; MMotionR input; MMotionL input
function output= fcn(Gait_phaseR, Gait_phaseL, STOPR, STOPL, MMotionR, MMotionL)
     output = [Gait_phaseR; Gait_phaseL; STOPR; STOPL; MMotionR; MMotionL];
end

== stateflow chart train_detection/RIGHT_LEG1/Pos and Vel normalized/Chart ==
  settings: updateMethod=DISCRETE  sampleTime=0.01
  state Expect_Vel_Max
    entry: valid_ang_min = 1;
    during:
    valid_vel_max = 0;
    valid_vel_min = 0;
    valid_ang_max = 0;
    valid_ang_min = 0;
  state Expect_Ang_Max
    entry: valid_vel_max = 1;
    during:
    valid_vel_max = 0;
    valid_vel_min = 0;
    valid_ang_max = 0;
    valid_ang_min = 0;
  state Resync
    valid_vel_max = 0;
    valid_vel_min = 0;
    valid_ang_max = 0;
    valid_ang_min = 0;
  state Expect_Vel_Min
    entry: valid_ang_max = 1;
    during:
    valid_vel_max = 0;
    valid_vel_min = 0;
    valid_ang_max = 0;
    valid_ang_min = 0;
  state Expect_Ang_Min
    entry: valid_vel_min = 1;
    during:
    valid_vel_max = 0;
    valid_vel_min = 0;
    valid_ang_max = 0;
    valid_ang_min = 0;
  Expect_Vel_Max -> Expect_Ang_Max [order 1] : [vel_max && after(Tmin, tick) && before(Tmax, tick) && vel > 0]
  Resync -> Expect_Ang_Max [order 1] : [vel_max && vel > 0]
  Expect_Vel_Max -> Resync [order 2] : [after(Tmax, tick)]
  Expect_Ang_Max -> Resync [order 2] : [after(Tmax, tick)]
  Expect_Ang_Max -> Expect_Vel_Min [order 1] : [ang_max && after(Tmin, tick) && before(Tmax, tick) && angle > 0]
  Expect_Ang_Min -> Expect_Vel_Max [order 2] : [ang_min && after(Tmin, tick) && before(Tmax, tick) && angle < 0]
  Resync -> Expect_Vel_Max [order 3] : [ang_min && angle < 0]
  Expect_Vel_Min -> Resync [order 1] : [after(Tmax, tick)]
  (default) -> Resync : {valid_vel_max = 0;
      | valid_vel_min = 0;
      | valid_ang_max = 0;
      | valid_ang_min = 0;}
  Resync -> Expect_Vel_Min [order 4] : [ang_max && angle > 0]
  Expect_Ang_Min -> Resync [order 1] : [after(Tmax, tick)]
  Resync -> Expect_Ang_Min [order 2] : [vel_min && vel < 0]
  Expect_Vel_Min -> Expect_Ang_Min [order 2] : [vel_min && after(Tmin, tick) && before(Tmax, tick) && vel < 0]
  data: ang_max input; vel_min input; vel_max input; ang_min input; valid_vel_max output; valid_vel_min output; valid_ang_max output; valid_ang_min output; Tmin local double =0; Tmax local double =60; vel input; angle input

== matlab function train_detection/IMUs/Kalman_Filter_R ==
  data: y input; x_hat output
function x_hat = kalman_hip(y)
% y: measured angle (scalar)
% x_hat: [theta_hat; theta_dot_hat]

persistent A C Q R P x
persistent initialized

Ts = 0.01; % sample time

if isempty(initialized)
    A = [1 Ts; 0 1];
    C = [1 0];

    % Tune these:
    Q = [1e-6      0;
        0      5e-3];   % more process noise on velocity state
    R = 9e-4;            % measurement noise variance (rad^2)

    P = eye(2);        % initial covariance
    x = [0; 0];        % initial state estimate
    initialized = true;
end

% Prediction
x_pred = A * x;
P_pred = A * P * A' + Q;

% Innovation
y_pred = C * x_pred;
e = y - y_pred;  % innovation

S = C * P_pred * C' + R;
K = P_pred * C' / S;  % Kalman gain (2x1)

% Update
x = x_pred + K * e;
P = (eye(2) - K * C) * P_pred;

x_hat = x;

== stateflow chart train_detection/LEFT LEG/Pos and Vel normalized/Chart ==
  settings: updateMethod=DISCRETE  sampleTime=0.01
  state Expect_Vel_Max
    entry: valid_ang_min = 1;
    during:
    valid_vel_max = 0;
    valid_vel_min = 0;
    valid_ang_max = 0;
    valid_ang_min = 0;
  state Expect_Ang_Max
    entry: valid_vel_max = 1;
    during:
    valid_vel_max = 0;
    valid_vel_min = 0;
    valid_ang_max = 0;
    valid_ang_min = 0;
  state Resync
    valid_vel_max = 0;
    valid_vel_min = 0;
    valid_ang_max = 0;
    valid_ang_min = 0;
  state Expect_Vel_Min
    entry: valid_ang_max = 1;
    during:
    valid_vel_max = 0;
    valid_vel_min = 0;
    valid_ang_max = 0;
    valid_ang_min = 0;
  state Expect_Ang_Min
    entry: valid_vel_min = 1;
    during:
    valid_vel_max = 0;
    valid_vel_min = 0;
    valid_ang_max = 0;
    valid_ang_min = 0;
  Expect_Vel_Max -> Expect_Ang_Max [order 1] : [vel_max && after(Tmin, tick) && before(Tmax, tick) && vel > 0]
  Resync -> Expect_Ang_Max [order 1] : [vel_max && vel > 0]
  Expect_Vel_Max -> Resync [order 2] : [after(Tmax, tick)]
  Expect_Ang_Max -> Resync [order 2] : [after(Tmax, tick)]
  Expect_Ang_Max -> Expect_Vel_Min [order 1] : [ang_max && after(Tmin, tick) && before(Tmax, tick) && angle > 0]
  Expect_Ang_Min -> Expect_Vel_Max [order 2] : [ang_min && after(Tmin, tick) && before(Tmax, tick) && angle < 0]
  Resync -> Expect_Vel_Max [order 3] : [ang_min && angle < 0]
  Expect_Vel_Min -> Resync [order 1] : [after(Tmax, tick)]
  (default) -> Resync : {valid_vel_max = 0;
      | valid_vel_min = 0;
      | valid_ang_max = 0;
      | valid_ang_min = 0;}
  Resync -> Expect_Vel_Min [order 4] : [ang_max && angle > 0]
  Expect_Ang_Min -> Resync [order 1] : [after(Tmax, tick)]
  Resync -> Expect_Ang_Min [order 2] : [vel_min && vel < 0]
  Expect_Vel_Min -> Expect_Ang_Min [order 2] : [vel_min && after(Tmin, tick) && before(Tmax, tick) && vel < 0]
  data: ang_max input; vel_min input; vel_max input; ang_min input; valid_vel_max output; valid_vel_min output; valid_ang_max output; valid_ang_min output; Tmin local double =0; Tmax local double =60; vel input; angle input

== matlab function train_detection/IMUs/MATLAB Function2 ==
  data: i input; y output; data input
function y = imuPlayback(i, data)
%#codegen
% imuData must be defined as a Simulink.Parameter in the base workspace.
% Example: imuData = Simulink.Parameter(yourIMUArray);

% y will be a 1x4 row vector
if i+1 <= size(data,1)
    y = data(i+1,:);      % pick row i
else
    y = data(end,:);    % after end, hold last value
end

end
